simulink model "iliad_ctrl"  (R2018b)
settings: Solver=FixedStepAuto  StartTime=0.0  StopTime=inf  FixedStep=0.01  RelTol=1e-3
values from neighbouring files (symbols this model uses):
  max_output_len = 4000    [iliad_init.m]    (also in iliad_test_init.m)
  pos_threshold = 0.1    [iliad_init.m]    (also in iliad_test_init.m)
  q_left_init = [0.1, 0.1, 0.1, 0, 0,  1, -1.5]'    [iliad_init.m]    (also in iliad_test_init.m)
  q_right_init = [0.1, 0.1, 0.1, 0, 0, -1,    0]'    [iliad_init.m]    (also in iliad_test_init.m)
  t_prova = [300,300;            300,300;            800,800;            800,800;            800,800]    [iliad_init.m]    (also in iliad_test_init.m)
libraries: robotlib x10, realtime_pacer_lib x2
settings Model: Creator=ed  LastModifiedBy=ed

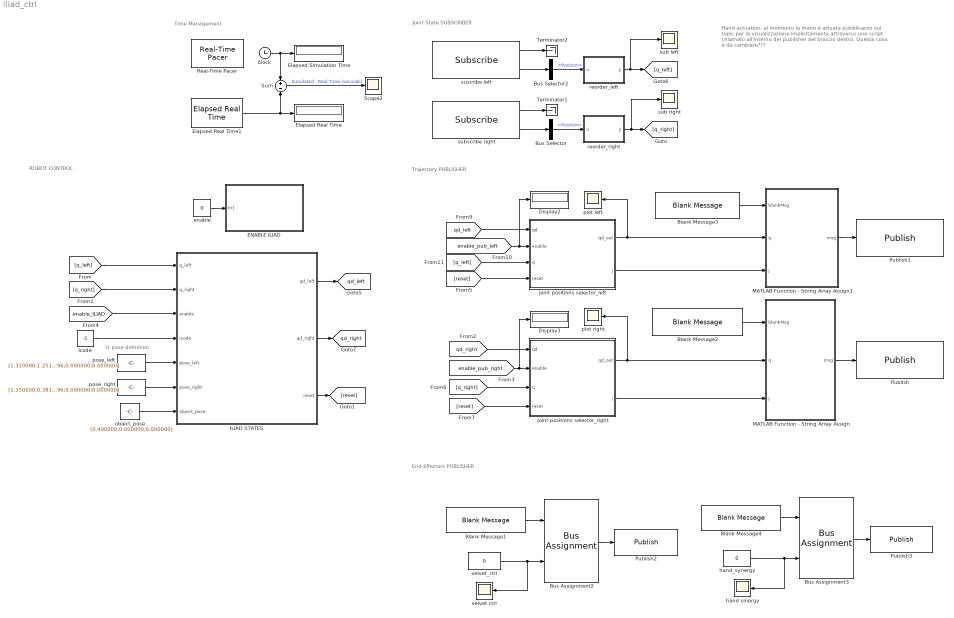
== system iliad_ctrl ==
  note: Hand actuation:
      | al momento la mano è attuata pubblicanto sul topic per la visualizzazione implicitamente attraverso uno script chiamato all'interno del publisher del braccio destro.
      | Questa cosa è da cambiare???
  note: I1 pose definition
  note: ROBOT CONTROL
  note: Time Management
  note: Joint State SUBSCRIBER
  note: Trajectory PUBLISHER
  note: End-Effectors PUBLISHER
  Blank Message1 : robotlib/Blank Message  messageClass=Message  entityType=std_msgs/Float64  messageType=std_msgs/Float64  SampleTime=inf
      settings: SourceProductBaseCode=RO
  Blank Message2 : robotlib/Blank Message  messageClass=Message  entityType=trajectory_msgs/JointTrajectory  messageType=trajectory_msgs/JointTrajectory  SampleTime=-1
      settings: SourceProductBaseCode=RO
  Blank Message3 : robotlib/Blank Message  messageClass=Message  entityType=trajectory_msgs/JointTrajectory  messageType=trajectory_msgs/JointTrajectory  SampleTime=-1
      settings: SourceProductBaseCode=RO
  Blank Message4 : robotlib/Blank Message  messageClass=Message  entityType=std_msgs/Float64  messageType=std_msgs/Float64  SampleTime=inf
      settings: SourceProductBaseCode=RO
  Bus Assignment2 : BusAssignment  AssignedSignals=Data
  Bus Assignment3 : BusAssignment  AssignedSignals=Data
  Bus Selector : BusSelector  OutputSignals=Position
  Bus Selector2 : BusSelector  OutputSignals=Position
  Clock : Clock
  Display2 : Display
  Display3 : Display
  ENABLE ILIAD : Subsystem
  Elapsed Real Time : Display
      settings: Decimation=2
  Elapsed Real Time1 : realtime_pacer_lib/Elapsed Real Time
  Elapsed Simulation Time : Display
      settings: Decimation=2
  ILIAD STATES : Stateflow chart  TreatAsAtomicUnit=on
  Icode : Constant  Value=-1
  MATLAB Function - String Array Assign : MATLAB Function  TreatAsAtomicUnit=on
  MATLAB Function - String Array Assign1 : MATLAB Function  TreatAsAtomicUnit=on
  Publish : robotlib/Publish  topicSource=Specify your own  topic=/right_arm/command_aux  messageType=trajectory_msgs/JointTrajectory  messageQueueLength=1
      settings: SourceProductBaseCode=RO
  Publish1 : robotlib/Publish  topicSource=Specify your own  topic=/left_arm/command_aux  messageType=trajectory_msgs/JointTrajectory  messageQueueLength=1
      settings: SourceProductBaseCode=RO
  Publish2 : robotlib/Publish  topicSource=Select from ROS network  topic=/velvet_cmd  messageType=std_msgs/Float64  messageQueueLength=1
      settings: SourceProductBaseCode=RO
  Publish3 : robotlib/Publish  topicSource=Select from ROS network  topic=/hand_cmd  messageType=std_msgs/Float64  messageQueueLength=1
      settings: SourceProductBaseCode=RO
  Real-Time Pacer : realtime_pacer_lib/Real-Time Pacer  simTimePerRealTime=1
  Scope2 : Scope
  Sum : Sum  Inputs=+|-
  Terminator1 : Terminator
  Terminator2 : Terminator
  enable : Constant  Value=0
  "hand sinergy " : Scope
  hand_synergy : Constant  Value=0
  joint positions selector_left : MATLAB Function  TreatAsAtomicUnit=on
  joint positions selector_right : MATLAB Function  TreatAsAtomicUnit=on
  object_pose : Constant  Value=[0.400000;0.000000;0.000000]
  plot left : Scope
  plot right : Scope
  pose_left : Constant  Value=[1.310000;1.251000;0.800000;1.570796;0.000000;0.000000]
  pose_right : Constant  Value=[1.350000;0.381000;0.800000;1.570796;0.000000;0.000000]
  reorder_left : MATLAB Function  TreatAsAtomicUnit=on
  reorder_right : MATLAB Function  TreatAsAtomicUnit=on
  sub left : Scope
  sub right : Scope
  subscribe right : robotlib/Subscribe  topicSource=Specify your own  topic=/right_arm/joint_states  messageType=sensor_msgs/JointState  sampleTime=-1  messageQueueLength=1
      settings: SourceProductBaseCode=RO
  suscribe left : robotlib/Subscribe  topicSource=Specify your own  topic=/left_arm/joint_states  messageType=sensor_msgs/JointState  sampleTime=-1  messageQueueLength=1
      settings: SourceProductBaseCode=RO
  "velvet ctrl " : Scope
  velvet_ctrl : Constant  Value=0
  tag scope: qd_left=global, qd_right=global
  wires:
  Sum/1 -> Scope2/1  "Simulated - Real Time (seconds)"
  Elapsed Real Time1/1 -> Sum/2, Elapsed Real Time/1
  Clock/1 -> Sum/1, Elapsed Simulation Time/1
  subscribe right/1 -> Terminator1/1
  suscribe left/2 -> Bus Selector2/1
  Bus Selector/1 -> reorder_right/1(u)  "<Position>"
  subscribe right/2 -> Bus Selector/1
  [q_right] -> joint positions selector_right/3(q)
  joint positions selector_left/1(qd_out) -> plot left/1, MATLAB Function - String Array Assign1/2(q)
  [q_left] -> joint positions selector_left/3(q)
  [qd_left] -> joint positions selector_left/1(qd)
  [qd_right] -> joint positions selector_right/1(qd)
  [enable_pub_right] -> Display3/1, joint positions selector_right/2(enable)
  [enable_pub_left] -> joint positions selector_left/2(enable), Display2/1
  [q_left] -> ILIAD STATES/1(q_left)
  [q_right] -> ILIAD STATES/2(q_right)
  reorder_right/1(y) -> [q_right], sub right/1
  Bus Selector2/1 -> reorder_left/1(u)  "<Position>"
  reorder_left/1(y) -> [q_left], sub left/1
  suscribe left/1 -> Terminator2/1
  [enable_ILIAD] -> ILIAD STATES/3(enable)
  ILIAD STATES/2(qd_right) -> [qd_right]
  enable/1 -> ENABLE ILIAD/1(In1)
  ILIAD STATES/1(qd_left) -> [qd_left]
  [reset] -> joint positions selector_right/4(reset)
  [reset] -> joint positions selector_left/4(reset)
  ILIAD STATES/3(reset) -> [reset]
  pose_left/1 -> ILIAD STATES/5(pose_left)
  pose_right/1 -> ILIAD STATES/6(pose_right)
  Icode/1 -> ILIAD STATES/4(Icode)
  joint positions selector_right/1(qd_out) -> plot right/1, MATLAB Function - String Array Assign/2(q)
  MATLAB Function - String Array Assign1/1(msg) -> Publish1/1
  Blank Message3/1 -> MATLAB Function - String Array Assign1/1(blankMsg)
  MATLAB Function - String Array Assign/1(msg) -> Publish/1
  Blank Message2/1 -> MATLAB Function - String Array Assign/1(blankMsg)
  object_pose/1 -> ILIAD STATES/7(object_pose)
  joint positions selector_right/2(j) -> MATLAB Function - String Array Assign/3(j)
  joint positions selector_left/2(j) -> MATLAB Function - String Array Assign1/3(j)
  velvet_ctrl/1 -> "velvet ctrl "/1, Bus Assignment2/2
  Bus Assignment2/1 -> Publish2/1
  Blank Message1/1 -> Bus Assignment2/1
  Bus Assignment3/1 -> Publish3/1
  hand_synergy/1 -> "hand sinergy "/1, Bus Assignment3/2
  Blank Message4/1 -> Bus Assignment3/1

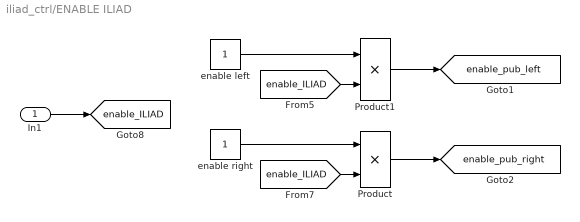
== system iliad_ctrl/ENABLE ILIAD ==
  In1 : Inport
  Product : Product
  Product1 : Product
  enable left : Constant
  enable right : Constant
  tag scope: enable_ILIAD=global, enable_pub_left=global, enable_pub_right=global
  wires:
  enable left/1 -> Product1/1
  Product/1 -> [enable_pub_right]
  Product1/1 -> [enable_pub_left]
  In1/1 -> [enable_ILIAD]
  enable right/1 -> Product/1
  [enable_ILIAD] -> Product1/2
  [enable_ILIAD] -> Product/2

== matlab function iliad_ctrl/joint positions selector_right ==
  data: qd input; enable input; qd_out output; j output; q input; reset input
function [qd_out, j] = publisher_(qd, enable, q, reset)
%% 
%qd_out = points to be send to the robot
%qd = entire trajectory generated by reverse priority
% enable = equal to 1 once a trajectpry qd has been generated by rev
% priority
%%
% if qd has been generated, this function selects consecutive joint
% positions along the trajectory qd to be send to the robot
persistent count 

if (isempty(count))
    count = 1;
end

if reset
    count = 1;
end

% manages arm joints
if (enable == 1)  % publish reference joint
   if (count > size(qd, 2))
       count =  size(qd, 2);
   end
   qd_out = qd(:, count);
   count = count + 1;
else  % publish robot current joint -> constant
    qd_out = q;
end

j = count;

end

== matlab function iliad_ctrl/reorder_right ==
  data: u input; y output
function y = reorder(u)
%this function reorder joint position readings 
y = u(1:7);
y(3) = u(7);
for i = 4 : 7
    y(i) = u(i-1);
end

end

== matlab function iliad_ctrl/reorder_left ==
  data: u input; y output
function y = reorder(u)
%this function reorder joint position readings 
y = u(1:7);
y(3) = u(7);
for i = 4 : 7
    y(i) = u(i-1);
end

end

== matlab function iliad_ctrl/MATLAB Function - String Array Assign ==
  data: blankMsg input; msg output Bus: SL_Bus_iliad_ctrl_trajectory_msgs_JointTrajectory; q input; j input
function msg = stringArrayAssign(blankMsg,q,j)
% stringArrayAssign - Assign a string array in a ROS message
%
%  blankMsg (input): A bus for a 'sensor_msgs/JointState' message. This is 
%      used to initialize the output.
%  msg (output): A bus for a 'sensor_msgs/JointState' message message, with 
%      Name field set to a string array.
%
%   Copyright 2015 The MathWorks, Inc.

%#codegen

% Note: The datatype of 'msg' has been explicitly set to the appropriate 
% Simulink bus type ("SL_Bus_robotROSMessageUsageExample_sensor_msgs_JointState"). 
%
% If the model name is changed, the datatype needs to be changed as well:
%   1) Click "Edit Data" in the Editor toolstrip to open "Ports and Data Manager"
%   2) Select "msg". From the "Type" dropdown, select "--- Refresh data types ---"
%   3) Set datatype to "Bus: SL_Bus_<modelname>_sensor_msgs_JointState"

strArrayToAssign = {'right_arm_a1_joint',...
                    'right_arm_a2_joint',...
                    'right_arm_e1_joint',...
                    'right_arm_a3_joint',...
                    'right_arm_a4_joint',...
                    'right_arm_a5_joint',...
                    'right_arm_a6_joint'};
msg = blankMsg;

% Set the number of strings in the string array.
% msg (sensor_msgs/JointState) includes the following fields
%           Name : array of std_msgs/String (string array)
%   Name_SL_Info : struct with fields CurrentLength, ReceivedLength
numStringsInArray = length(strArrayToAssign);
msg.JointNames_SL_Info.CurrentLength = uint32(numStringsInArray);
msg.Points_SL_Info.CurrentLength = uint32(1);

% Set the individual strings in the array
for idx = 1 : numStringsInArray
    str = strArrayToAssign{idx};
    strLength = length(str);
    msg.JointNames(idx).Data(1:strLength) = uint8(str);
    msg.JointNames(idx).Data_SL_Info.CurrentLength = uint32(strLength);
end
msg.Points(1).Positions(1:length(q)) = q;
msg.Points(1).Positions_SL_Info.CurrentLength = uint32(length(q));
msg.Points(1).TimeFromStart.Sec = 0;
msg.Points(1).TimeFromStart.Nsec = 5000000;

msg.Header.Seq = uint32(j);

== stateflow chart iliad_ctrl/ILIAD STATES ==
  state Go2Waypoint
    % execute waypoints received from dual manipulation
    en:
    coder.extrinsic('go2pose');
    coder.extrinsic('check_end_move');
    coder.extrinsic('retrieve_mov');
    % default variables, initialization
    reset = 1;
    change_state = 0;
    changing = 0;
    scale_traj = 1;
    % retrieve next waypoint
    [manipulation_mov, change_state] = retrieve_mov();
    if change_state == 0 % reach waypoint
    [qd_left, qd_right] = go2pose(q_curr_left, q_curr_right,...
    manipulation_mov(1:6), manipulation_mov(7:12),...
    t_prova, max_output_len, scale_traj);
    elseif change_state == 1 % end of the movement, go home
    changing = 1; reset = 0;
    else % change_state == 2, stay still
    changing = 2; reset = 0;
    end
    %% ------------------------------------------------------------ %%
    du:
    reset = 0;
    flag_state = check_end_move(qd_left, qd_right, q_left, q_right,...
    max_output_len, pos_threshold);
    %% ------------------------------------------------------------ %%
    ex:
    q_curr_left = qd_left(:, end);
    q_curr_right = qd_right(:, end);
  state homing
    % send the robot in the home position
    en:
    coder.extrinsic('homing');
    coder.extrinsic('check_end_move');
    reset = 1;
    scale_traj = 0;
    [qd_left, qd_right] = homing(q_curr_left, q_curr_right,...
    t_prova, max_output_len, scale_traj);
    %% ------------------------------------------------------------ %%
    du:
    reset = 0;
    flag_state = check_end_move(qd_left, qd_right, q_left, q_right,...
    max_output_len, pos_threshold);
    %% ------------------------------------------------------------ %%
    ex:
    q_curr_left = qd_left(:, end);
    q_curr_right = qd_right(:, end);
  state init
    en:
    qd_left   = repmat(q_left_init,   1, max_output_len );
    qd_right = repmat(q_right_init, 1, max_output_len );
    ex:
    q_curr_left = qd_left(:, end);
    q_curr_right = qd_right(:, end);
  state Idle
    en:
    coder.extrinsic('idle_Icode');
    % set the Icode to -1
    idle_Icode();
  state Go2Pose
    % send the robot to a position defined as input of the state machine,
    % you can specify it from command line using the Icode
    en:
    coder.extrinsic('go2pose');
    coder.extrinsic('check_end_move');
    reset = 1;
    scale_traj = 0;
    %%
    [qd_left, qd_right] = go2pose(q_curr_left, q_curr_right,...
    pose_left, pose_right,...
    t_prova, max_output_len, scale_traj);
    %% ------------------------------------------------------------ %%
    du:
    reset = 0;
    flag_state = check_end_move(qd_left, qd_right, q_left, q_right,...
    max_output_len, pos_threshold);
    %% ------------------------------------------------------------ %%
    ex:
    q_curr_left = qd_left(:, end);
    q_curr_right = qd_right(:, end);
  state MakeMovement
    % make a default movement based on the object position, this is
    % more like a test than a true capability for the robot
    en:
    coder.extrinsic('go2pose');
    coder.extrinsic('check_end_move');
    coder.extrinsic('object2waypoint');
    reset = 1;
    scale_traj = 1;
    %%
    [wp_l, wp_r] = object2waypoint(object_pose);
    [qd_left, qd_right] = go2pose(q_curr_left, q_curr_right, ...
    wp_l, wp_r,...
    t_prova, max_output_len, scale_traj);
    %% ------------------------------------------------------------ %%
    du:
    reset = 0;
    flag_state = check_end_move(qd_left, qd_right, q_left, q_right,...
    max_output_len, pos_threshold);
    %% ------------------------------------------------------------ %%
    ex:
    q_curr_left = qd_left(:, end);
    q_curr_right = qd_right(:, end);
  Go2Waypoint -> Go2Waypoint [order 1] : [flag_state == 1]
      | {flag_state = 0}
  Go2Waypoint -> homing [order 2] : [changing == 1]
  (default) -> init
  init -> homing : [enable == 1]{flag_state = 0}
  Go2Waypoint -> Idle [order 3] : [changing ==2]
  homing -> Idle : [flag_state == 1]
      | {flag_state = 0}
  Idle -> homing [order 1] : [Icode == 0]
  Idle -> Go2Waypoint [order 4] : [Icode == 3]
  Idle -> MakeMovement [order 2] : [Icode == 2]
  Idle -> Go2Pose [order 3] : [Icode == 1]
  Go2Pose -> Idle : [flag_state == 1]
      | {flag_state = 0}
  MakeMovement -> Idle : [flag_state == 1]
      | {flag_state = 0}
  data: t_prova parameter; max_output_len parameter; q_left input size=[7 1]; q_right input size=[7 1]; enable input; Icode input; qd_left output size=[7 max_output_len]; qd_right output size=[7 max_output_len]; q_right_init parameter; q_curr_right local; q_curr_left local; pose_left input; reset output; pose_right input; flag_state local double size=1 =0; pos_threshold parameter; q_left_init parameter; object_pose input; wp_r local; wp_l local; manipulation_mov local; change_state local; changing local; scale_traj local

== matlab function iliad_ctrl/joint positions selector_left ==
  data: qd input; enable input; qd_out output; j output; q input; reset input
function [qd_out, j] = publisher_(qd, enable, q, reset)
%% 
%qd_out = points to be send to the robot
%qd = entire trajectory generated by reverse priority
% enable = equal to 1 once a trajectory qd has been generated by rev
% priority
%%
% if qd has been generated, this function selects consecutive joint
% positions along the trajectory qd to be send to the robot
persistent count 

if(isempty(count))
    count = 1;
end

if reset
    count = 1;
end

if (enable == 1)  % publish reference joint
   if (count > size(qd, 2))
       count =  size(qd, 2);
   end
   qd_out = qd(:, count);
   count = count + 1;
else  % publish robot current joint -> constant
    qd_out = q;
end
j = count;

end

== matlab function iliad_ctrl/MATLAB Function - String Array Assign1 ==
  data: blankMsg input; msg output Bus: SL_Bus_iliad_ctrl_trajectory_msgs_JointTrajectory; q input; j input
function msg = stringArrayAssign(blankMsg,q,j)
% stringArrayAssign - Assign a string array in a ROS message
%
%  blankMsg (input): A bus for a 'sensor_msgs/JointState' message. This is 
%      used to initialize the output.
%  msg (output): A bus for a 'sensor_msgs/JointState' message message, with 
%      Name field set to a string array.
%
%   Copyright 2015 The MathWorks, Inc.

%#codegen

% Note: The datatype of 'msg' has been explicitly set to the appropriate 
% Simulink bus type ("SL_Bus_robotROSMessageUsageExample_sensor_msgs_JointState"). 
%
% If the model name is changed, the datatype needs to be changed as well:
%   1) Click "Edit Data" in the Editor toolstrip to open "Ports and Data Manager"
%   2) Select "msg". From the "Type" dropdown, select "--- Refresh data types ---"
%   3) Set datatype to "Bus: SL_Bus_<modelname>_sensor_msgs_JointState"

strArrayToAssign = {'right_arm_a1_joint',...
                    'right_arm_a2_joint',...
                    'right_arm_e1_joint',...
                    'right_arm_a3_joint',...
                    'right_arm_a4_joint',...
                    'right_arm_a5_joint',...
                    'right_arm_a6_joint'};
msg = blankMsg;

% Set the number of strings in the string array.
% msg (sensor_msgs/JointState) includes the following fields
%           Name : array of std_msgs/String (string array)
%   Name_SL_Info : struct with fields CurrentLength, ReceivedLength
numStringsInArray = length(strArrayToAssign);
msg.JointNames_SL_Info.CurrentLength = uint32(numStringsInArray);
msg.Points_SL_Info.CurrentLength = uint32(1);

% Set the individual strings in the array
for idx = 1 : numStringsInArray
    str = strArrayToAssign{idx};
    strLength = length(str);
    msg.JointNames(idx).Data(1:strLength) = uint8(str);
    msg.JointNames(idx).Data_SL_Info.CurrentLength = uint32(strLength);
end
msg.Points(1).Positions(1:length(q)) = q;
msg.Points(1).Positions_SL_Info.CurrentLength = uint32(length(q));
msg.Points(1).TimeFromStart.Sec = 0;
msg.Points(1).TimeFromStart.Nsec = 5000000;

msg.Header.Seq = uint32(j);
